simulink model "closed_base_1ph"  (R2024a)
settings: Solver=VariableStepAuto  StartTime=0.0  StopTime=20  RelTol=1e-3
libraries: spsSeriesRLCBranchLib x8, spsVoltageMeasurementLib x5, spsBreakerLib x2, spsDiodeLib x1, spsIGBTDiodeLib x1, spsPLLLib x1, spsPVArrayLib x1, spsPWMGenerator2LevelLib x1, spsPWMGeneratorDCDCLib x1, spsUniversalBridgeLib x1, sps_lib x1
settings Model: Creator=megha  LastModifiedBy=megha

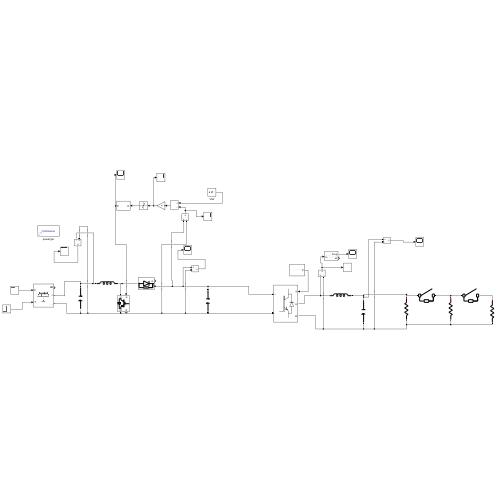
[thumbnail: Simulink's stored preview of the top-level diagram]
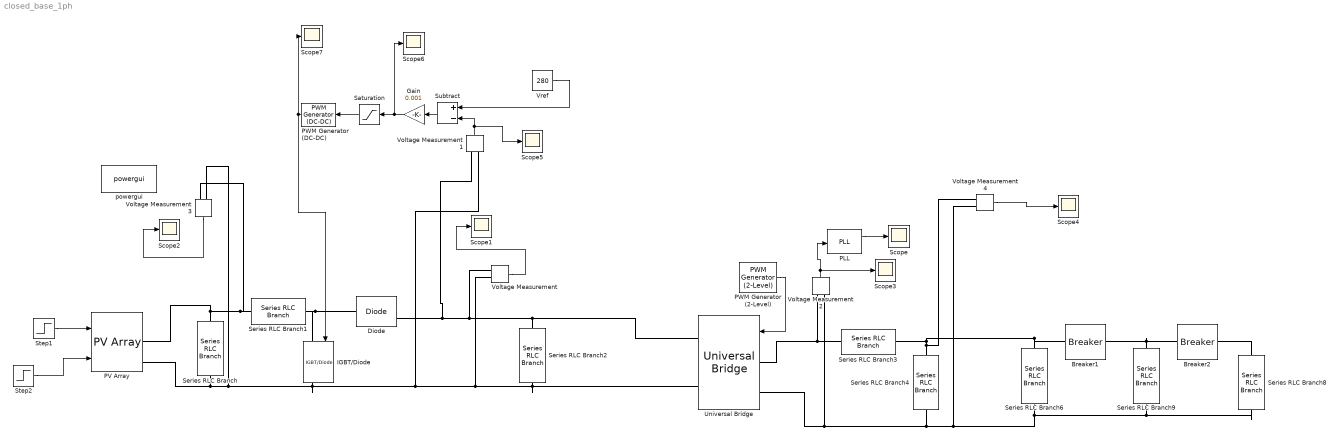
== system closed_base_1ph ==
  Breaker1 : spsBreakerLib/Breaker  InitialState=0  SwitchingTimes="[5  10]"  External=off  BreakerResistance=0.01  SnubberResistance=1e6  SnubberCapacitance=inf  Measurements=None  MoreParameters=on  NoBreakLoop=off
  Breaker2 : spsBreakerLib/Breaker  InitialState=0  SwitchingTimes=[0 5]  External=off  BreakerResistance=0.01  SnubberResistance=1e6  SnubberCapacitance=inf  Measurements=None  MoreParameters=on  NoBreakLoop=off
  Diode : spsDiodeLib/Diode  Ron=0.001  Lon=0  Vf=0.8  IC=0  UseSnubber=0  Rs=500  Cs=250e-9  Measurements=on
  Gain : Gain  Gain=0.001
  IGBT/Diode : spsIGBTDiodeLib/IGBT//Diode  Ron=1e-3  Rs=1e5  Cs=inf  Measurements=on
  PLL : spsPLLLib/PLL  Fmin=45  Par_Init=[0, 60]  ParK=[180, 3200, 1]  TcD=1e-4  MaxRateChangeFreq=12  FilterCutOffFreq=25  Ts=0  AGC=on
      settings: LibrarySourceBlock=sps_lib/Control/PLL
  PV Array : spsPVArrayLib/PV Array  Npar=40  Nser=4  PlotType=array @ 1000 W/m2 & specified temperatures  S_vec="[ 1000  500  100 ]"  Temp_C_vec="[ 45 25  ]"  ModuleName=User-defined  PlotWhenSelected=off  Pm=213.15  Ncell=60  Voc=36.3  Isc=7.84  Vm=29  Im=7.35  beta_Voc_pc=-0.36099  alpha_Isc_pc=0.102  beta_Voc=-0.13104  alpha_Isc=0.0079968  IL=7.8654  I0=2.9273e-10  nI=0.98119  Rsh=313.0553  Rs=0.39381  RobustModel=off  RobustCellTemperature=313.3991  BAL=on  Tc=1e-6  Tfilter=5e-5
  PWM Generator (2-Level) : spsPWMGenerator2LevelLib/PWM Generator (2-Level)  ModulatorType=Single-phase full-bridge (4 pulses)  ModulatorMode=Unsynchronized  Fc=27*60  Pc=90  nF=27  MinMax="[ -1  1 ]"  SamplingTechnique=Natural  ModulatingSignals=on  m=1  Freq=60  Phase=0  Ts=0  ShowCarrierOutport=off
  PWM Generator (DC-DC) : spsPWMGeneratorDCDCLib/PWM Generator (DC-DC)  Fsw=1500  Ts=0
  Saturation : Saturate  UpperLimit=1  LowerLimit=0
  Scope{,1..7} (8 alike) : Scope
  Series RLC Branch : spsSeriesRLCBranchLib/Series RLC Branch  LConnTagsString=__new0  RConnTagsString=__new0  BranchType=C  Resistance=1  Inductance=1e-3  SetiL0=off  InitialCurrent=0  Capacitance=0.006  Setx0=off  InitialVoltage=0  Measurements=None
  Series RLC Branch1 : spsSeriesRLCBranchLib/Series RLC Branch  LConnTagsString=__new0  RConnTagsString=__new0  BranchType=L  Resistance=1  Inductance=0.02  SetiL0=off  InitialCurrent=0  Capacitance=1e-6  Setx0=off  InitialVoltage=0  Measurements=None
  Series RLC Branch2 : spsSeriesRLCBranchLib/Series RLC Branch  LConnTagsString=__new0  RConnTagsString=__new0  BranchType=C  Resistance=1  Inductance=1e-3  SetiL0=off  InitialCurrent=0  Capacitance=0.006  Setx0=off  InitialVoltage=0  Measurements=None
  Series RLC Branch3 : spsSeriesRLCBranchLib/Series RLC Branch  LConnTagsString=__new0  RConnTagsString=__new0  BranchType=L  Resistance=1  Inductance=0.02  SetiL0=off  InitialCurrent=0  Capacitance=1e-6  Setx0=off  InitialVoltage=0  Measurements=None
  Series RLC Branch4 : spsSeriesRLCBranchLib/Series RLC Branch  LConnTagsString=__new0  RConnTagsString=__new0  BranchType=C  Resistance=1  Inductance=1e-3  SetiL0=off  InitialCurrent=0  Capacitance=0.006  Setx0=off  InitialVoltage=0  Measurements=None
  Series RLC Branch6 : spsSeriesRLCBranchLib/Series RLC Branch  LConnTagsString=__new0  RConnTagsString=__new0  BranchType=R  Resistance=100  Inductance=1e-3  SetiL0=off  InitialCurrent=0  Capacitance=1e-6  Setx0=off  InitialVoltage=0  Measurements=None
  Series RLC Branch8 : spsSeriesRLCBranchLib/Series RLC Branch  LConnTagsString=__new0  RConnTagsString=__new0  BranchType=R  Resistance=60  Inductance=1e-3  SetiL0=off  InitialCurrent=0  Capacitance=1e-6  Setx0=off  InitialVoltage=0  Measurements=None
  Series RLC Branch9 : spsSeriesRLCBranchLib/Series RLC Branch  LConnTagsString=__new0  RConnTagsString=__new0  BranchType=R  Resistance=30  Inductance=0.005  SetiL0=off  InitialCurrent=0  Capacitance=1e-6  Setx0=off  InitialVoltage=0  Measurements=None
  Step1 : Step  Time=0.5  Before=1000  After=800  SampleTime=0
  Step2 : Step  Before=25  After=32  SampleTime=0
  Subtract : Sum  Inputs=+-
  Universal Bridge : spsUniversalBridgeLib/Universal Bridge  Arms=2  SnubberResistance=1e5  SnubberCapacitance=inf  Device=IGBT / Diodes  Ron=1e-3  Lon=0  ForwardVoltages="[  0  0  ]"  ForwardVoltage=0  GTOparameters=[ 10e-6 , 20e-6 ]  IGBTparameters=[ 1e-6 , 2e-6 ]  Measurements=None  Measurements_2=None  converterType=Rectifier
  Voltage Measurement{,1..4} (5 alike) : spsVoltageMeasurementLib/Voltage Measurement  PhasorSimulation=off  OutputType=Complex  PSBequivalent=0
  Vref : Constant  Value=280
  powergui : sps_lib/powergui  Priority=1  SimulationMode=Continuous  SampleTime=50e-6  frequency=60  Iterations=50  frequencyindice=0  Pbase=100e6  ErrMax=1e-4  UnitsV=kV  UnitsW=MW  buscounter=0  FunctionMessages=off  echomessages=off  EnableUseOfTLC=off  CurrentSourceSwitches=off  DisableSnubberDevices=off  DisableRonSwitches=off  DisableVfSwitches=off  DisplayEquations=off  AutomaticDiscreteSolvers=off  SolverType=Tustin/Backward Euler (TBE)  Interpol=off  ExternalGateDelay=off  methode=off  Ts=100  x0status=blocks  SPID=on  SwTol=0  HookPort=off  NonlinearTolerance=1e-4  nMaxIteration=100  ContinueOnMaxIteration=off  RestoreLinks=warning  ResistiveCurrentMeasurement=off  Frange=[0:2:500]  Ylog=off  Xlog=on  ShowGrid=off  save=off  variable=ZData  structure=0  ZoomFFT=off  StartTime=0.0  cycles=1  DisplayStyle=1  fundamental=60  FreqAxis=off  MaxFrequency=1000  frequencyindicesteady=1  RmsSteady=1  display=off
  wires:
  Voltage Measurement2/1 -> Scope3/1, PLL/1
  PWM Generator (2-Level)/1 -> Universal Bridge/1
  PLL/1 -> Scope/1
  Voltage Measurement/1 -> Scope1/1
  Voltage Measurement3/1 -> Scope2/1
  Voltage Measurement4/1 -> Scope4/1
  Voltage Measurement1/1 -> Scope5/1, Subtract/2
  Gain/1 -> Scope6/1, Saturation/1
  PWM Generator (DC-DC)/1 -> IGBT/Diode/1, Scope7/1
  Subtract/1 -> Gain/1
  Vref/1 -> Subtract/1
  Saturation/1 -> PWM Generator (DC-DC)/1
  Step2/1 -> PV Array/2
  Step1/1 -> PV Array/1
  connections:
  IGBT/Diode/RConn1 -- Universal Bridge/RConn2 -- Series RLC Branch2/RConn1 -- Voltage Measurement/LConn2 -- Voltage Measurement1/LConn2 -- Voltage Measurement3/LConn1 -- PV Array/RConn2 -- Series RLC Branch/RConn1
  Series RLC Branch9/RConn1 -- Series RLC Branch8/RConn1 -- Voltage Measurement2/LConn2 -- Universal Bridge/LConn2 -- Series RLC Branch4/RConn1 -- Voltage Measurement4/LConn2 -- Series RLC Branch6/RConn1
  Universal Bridge/RConn1 -- Voltage Measurement1/LConn1 -- Diode/RConn1 -- Voltage Measurement/LConn1 -- Series RLC Branch2/LConn1
  Voltage Measurement2/LConn1 -- Universal Bridge/LConn1 -- Series RLC Branch3/LConn1
  IGBT/Diode/LConn1 -- Series RLC Branch1/RConn1 -- Diode/LConn1
  PV Array/RConn1 -- Voltage Measurement3/LConn2 -- Series RLC Branch1/LConn1 -- Series RLC Branch/LConn1
  Series RLC Branch6/LConn1 -- Voltage Measurement4/LConn1 -- Series RLC Branch4/LConn1 -- Series RLC Branch3/RConn1 -- Breaker1/LConn1
  Series RLC Branch9/LConn1 -- Breaker1/RConn1 -- Breaker2/LConn1
  Breaker2/RConn1 -- Series RLC Branch8/LConn1
